simulink model "PitchHoldAndAirspeedHold"  (R2021b)
settings: Solver=VariableStepAuto  StartTime=0.0  StopTime=100  RelTol=1e-3
values from neighbouring files (symbols this model uses):
  alpha0 = 0.1824    [Glideslope.m]
  max_dev_elevator = 25 - trim_control_lo(1)    [Glideslope.m]
  max_dev_thrust = 19000 - trim_thrust_lo    [Glideslope.m]
  min_dev_elevator = -25 - trim_control_lo(1)    [Glideslope.m]
  min_dev_thrust = 1000 - trim_thrust_lo    [Glideslope.m]
  t0 = 10    [Glideslope.m]
  theta0 = 0.1824    [Glideslope.m]
  V_0 = 300    [Glideslope.m]
undefined symbols (not defined in the file or in its folder): coeff_x, coeff_y, magnitude, x0
libraries: slpidlib x3, cstblocks x1
settings Model: Creator=ddefu  LastModifiedBy=20181021

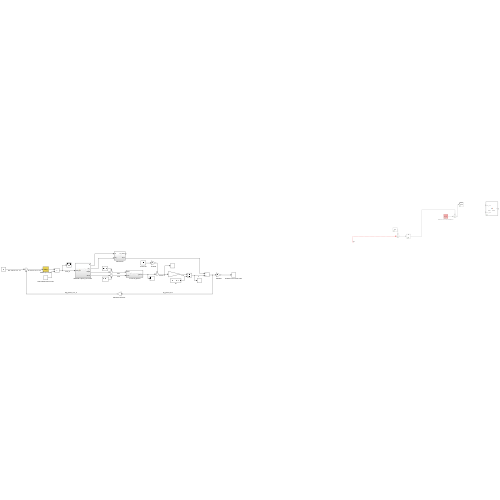
[thumbnail: Simulink's stored preview of the top-level diagram]
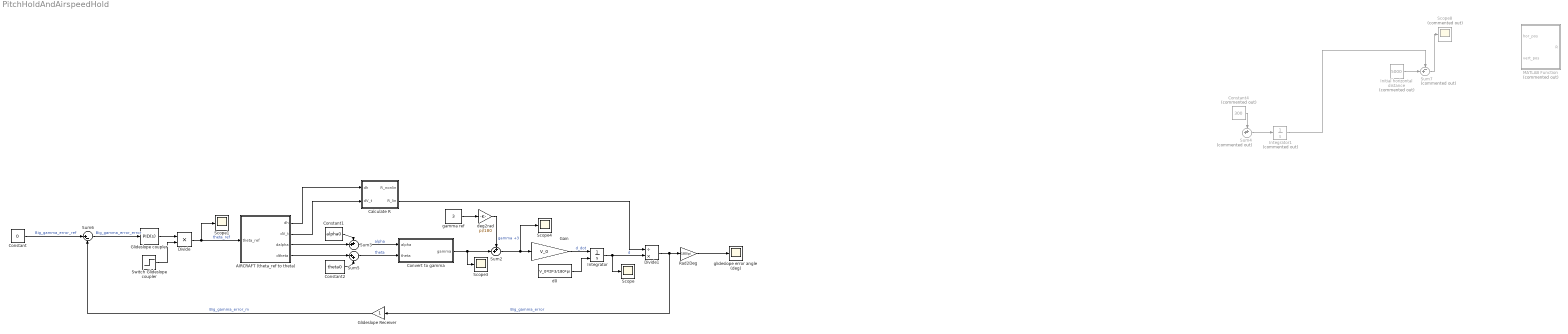
== system PitchHoldAndAirspeedHold ==
  AIRCRAFT (theta_ref to theta) : Subsystem
  Calculate R : Subsystem
  Constant : Constant  Value=0
  Constant1 : Constant  Value=alpha0
  Constant2 : Constant  Value=theta0
  Constant4 : Constant  Commented=on  Value=300
  Convert to gamma : Subsystem
  Divide : Product  Inputs=**
  Divide1 : Product  Inputs=/*
  Gain : Gain  Gain=V_0
  Glideslope Receiver : Gain
  Glideslope coupler : slpidlib/PID Controller  Controller=PID  Form=Parallel  TimeDomain=Continuous-time  UseExternalTs=off  SampleTime=-1  IntegratorMethod=Forward Euler  FilterMethod=Forward Euler  ControllerParametersSource=internal  P=100  I=10  D=0  UseFilter=on  N=100  TunerSelectOption=Transfer Function Based (PID Tuner App)  InitialConditionSource=internal  InitialConditionForIntegrator=0  InitialConditionForFilter=0  DifferentiatorICPrevScaledInput=0  ExternalReset=none  TrackingMode=off  Kt=1  LimitOutput=off  SatLimitsSource=internal  UpperSaturationLimit=inf  LowerSaturationLimit=-inf  LinearizeAsGain=on  AntiWindupMode=none  Kb=1  POutMin=[]  POutMax=[]  IOutMin=[]  IOutMax=[]  DOutMin=[]  DOutMax=[]  NOutMin=[]  NOutMax=[]  SumOutMin=[]  SumOutMax=[]  SaturationOutMin=[]  SaturationOutMax=[]  PParamMin=[]  PParamMax=[]  IParamMin=[]  IParamMax=[]  DParamMin=[]  DParamMax=[]  NParamMin=[]  NParamMax=[]  KbParamMin=[]  KbParamMax=[]  KtParamMin=[]  KtParamMax=[]  KbOutMin=[]  KbOutMax=[]  KtOutMin=[]  KtOutMax=[]  IntegratorOutMin=[]  IntegratorOutMax=[]  FilterOutMin=[]  FilterOutMax=[]  SumI1OutMin=[]  SumI1OutMax=[]  SumI2OutMin=[]  SumI2OutMax=[]  SumI3OutMin=[]  SumI3OutMax=[]  SumI4OutMin=[]  SumI4OutMax=[]  SumDOutMin=[]  SumDOutMax=[]  DifferentiatorOutMin=[]  DifferentiatorOutMax=[]  FilterDiffOutCoefMin=[]  FilterDiffOutCoefMax=[]  ReciprocalOutMin=[]  ReciprocalOutMax=[]  SumDenOutMin=[]  SumDenOutMax=[]  SumNumOutMin=[]  SumNumOutMax=[]  DivideOutMin=[]  DivideOutMax=[]  UdiffTsProdOutMin=[]  UdiffTsProdOutMax=[]  NTsProdOutMin=[]  NTsProdOutMax=[]  UintegralTsProdOutMin=[]  UintegralTsProdOutMax=[]  UngainTsProdOutMin=[]  UngainTsProdOutMax=[]  IntegratorContinuousStateAttributes=''  IntegratorStateMustResolveToSignalObject=off  IntegratorRTWStateStorageClass=Auto  FilterContinuousStateAttributes=''  FilterStateMustResolveToSignalObject=off  FilterRTWStateStorageClass=Auto  ParallelPVariant=InternalParameters  IdealPVariant=Disabled  IVariant=InternalParameters  DVariant=InternalParameters  IntegratorVariant=Continuous  SatVariant=Disabled  AWVariant=Passthrough  PCopyVariant=Disabled  TRVariant=Disabled  FdbkBlocksVariant=Forward  IdealPFdbkVariant=Disabled  SatFdbkVariant=Disabled  DerivativeFilterVariant=ContFilter  NVariant=InternalParameters  NCopyVariant=Disabled  FilterICVariant=InternalICsFilter  IntegratorICVariant=InternalICs  ExternalResetVariant=Disabled  TRSumVariant=Passthrough  SumFdbkVariant=Disabled  SumVariant=Sum_PID  TsampFilterVariant=InternalTs  TsampNgainVariant=Passthrough  TsampIntegralVariant=Passthrough  ExternalSaturationOutDataTypeStr=Inherit: Same as second input
  Initial horizontal distance : Constant  Commented=on  Value=5000
  Integrator : Integrator  InitialConditionSource=external
  Integrator1 : Integrator  Commented=on
  MATLAB Function : MATLAB Function  Commented=on  TreatAsAtomicUnit=on
  Rad2Deg : Gain  Gain=180/pi
  Scope{,1,3..4} (4 alike) : Scope
  Scope8 : Scope  Commented=on
  Sum2 : Sum  Inputs=++|
  Sum3 : Sum  Inputs=++|
  Sum4 : Sum  Commented=on  Inputs=++|
  Sum5 : Sum  Inputs=|++
  Sum6 : Sum  Inputs=|+-
  Sum7 : Sum  Commented=on  Inputs=-+|
  Switch Glideslope coupler : Step  Time=10  SampleTime=0
  d0 : Constant  Value=V_0*t0*3/180*pi
  deg2rad : Gain  Gain=pi/180
  gamma ref : Constant  Value=3
  glideslope error angle (deg) : Scope
  wires:
  Sum2/1 -> Scope4/1, Gain/1  "gamma +3"
  Gain/1 -> Integrator/1  "d_dot"
  Integrator/1 -> Divide1/2, Scope/1  "d"
  Convert to gamma/1(gamma) -> Sum2/2, Scope3/1
  Sum3/1 -> Convert to gamma/1(alpha)  "alpha"
  Constant1/1 -> Sum3/1
  Sum5/1 -> Convert to gamma/2(theta)  "theta"
  Divide1/1 -> Glideslope Receiver/1, Rad2Deg/1  "Big_gamma_error"
  Glideslope Receiver/1 -> Sum6/2  "Big_gamma_error_m"
  Constant/1 -> Sum6/1  "Big_gamma_error_ref"
  Sum6/1 -> Glideslope coupler/1  "Big_gamma_error_error"
  d0/1 -> Integrator/2
  Sum7/1 -> Scope8/1
  ? -> Sum4/2  "V_t"
  Integrator1/1 -> Sum7/1
  Constant4/1 -> Sum4/1
  Initial horizontal distance/1 -> Sum7/2
  Sum4/1 -> Integrator1/1
  Rad2Deg/1 -> glideslope error angle (deg)/1
  AIRCRAFT (theta_ref to theta)/1(dh) -> Calculate R/1(dh)
  AIRCRAFT (theta_ref to theta)/2(dV_t) -> Calculate R/2(dV_t)
  AIRCRAFT (theta_ref to theta)/3(dalpha) -> Sum3/2
  Switch Glideslope coupler/1 -> Divide/2
  Glideslope coupler/1 -> Divide/1
  Divide/1 -> Scope1/1, AIRCRAFT (theta_ref to theta)/1(theta_ref)  "theta_ref"
  Calculate R/2(R_lin) -> Divide1/1
  Constant2/1 -> Sum5/2
  AIRCRAFT (theta_ref to theta)/4(dtheta) -> Sum5/1
  gamma ref/1 -> deg2rad/1
  deg2rad/1 -> Sum2/1

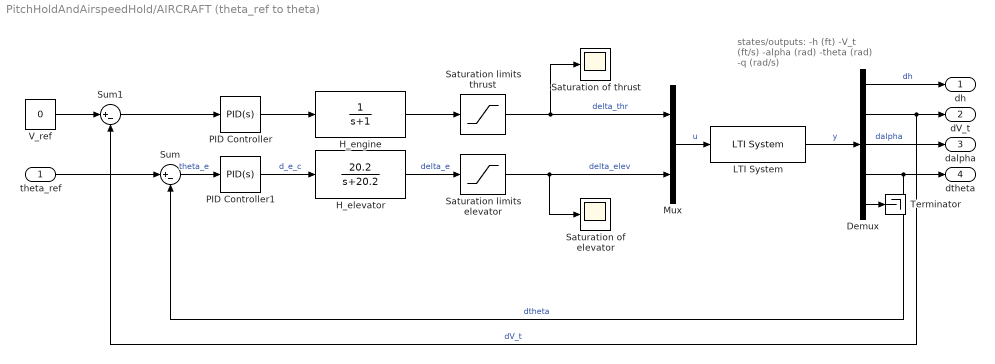
== system PitchHoldAndAirspeedHold/AIRCRAFT (theta_ref to theta) ==
  note: states/outputs:
      | -h (ft)
      | -V_t (ft/s)
      | -alpha (rad)
      | -theta (rad)
      | -q (rad/s)
  theta_ref : Inport
  Demux : Demux  Outputs=5
  H_elevator : TransferFcn  Numerator=[20.2]  Denominator=[1 20.2]
  H_engine : TransferFcn  Denominator=[1 1]
  LTI System : cstblocks/LTI System  sys=sys_reduced  IC=[0;0;0;0;0]
  Mux : Mux  Inputs=2
  PID Controller : slpidlib/PID Controller  Controller=PID  Form=Parallel  TimeDomain=Continuous-time  UseExternalTs=off  SampleTime=-1  IntegratorMethod=Forward Euler  FilterMethod=Forward Euler  ControllerParametersSource=internal  P=210  I=6  D=0  UseFilter=on  N=100  TunerSelectOption=Transfer Function Based (PID Tuner App)  InitialConditionSource=internal  InitialConditionForIntegrator=0  InitialConditionForFilter=0  DifferentiatorICPrevScaledInput=0  ExternalReset=none  TrackingMode=off  Kt=1  LimitOutput=off  SatLimitsSource=internal  UpperSaturationLimit=inf  LowerSaturationLimit=-inf  LinearizeAsGain=on  AntiWindupMode=none  Kb=1  POutMin=[]  POutMax=[]  IOutMin=[]  IOutMax=[]  DOutMin=[]  DOutMax=[]  NOutMin=[]  NOutMax=[]  SumOutMin=[]  SumOutMax=[]  SaturationOutMin=[]  SaturationOutMax=[]  PParamMin=[]  PParamMax=[]  IParamMin=[]  IParamMax=[]  DParamMin=[]  DParamMax=[]  NParamMin=[]  NParamMax=[]  KbParamMin=[]  KbParamMax=[]  KtParamMin=[]  KtParamMax=[]  KbOutMin=[]  KbOutMax=[]  KtOutMin=[]  KtOutMax=[]  IntegratorOutMin=[]  IntegratorOutMax=[]  FilterOutMin=[]  FilterOutMax=[]  SumI1OutMin=[]  SumI1OutMax=[]  SumI2OutMin=[]  SumI2OutMax=[]  SumI3OutMin=[]  SumI3OutMax=[]  SumI4OutMin=[]  SumI4OutMax=[]  SumDOutMin=[]  SumDOutMax=[]  DifferentiatorOutMin=[]  DifferentiatorOutMax=[]  FilterDiffOutCoefMin=[]  FilterDiffOutCoefMax=[]  ReciprocalOutMin=[]  ReciprocalOutMax=[]  SumDenOutMin=[]  SumDenOutMax=[]  SumNumOutMin=[]  SumNumOutMax=[]  DivideOutMin=[]  DivideOutMax=[]  UdiffTsProdOutMin=[]  UdiffTsProdOutMax=[]  NTsProdOutMin=[]  NTsProdOutMax=[]  UintegralTsProdOutMin=[]  UintegralTsProdOutMax=[]  UngainTsProdOutMin=[]  UngainTsProdOutMax=[]  IntegratorContinuousStateAttributes=''  IntegratorStateMustResolveToSignalObject=off  IntegratorRTWStateStorageClass=Auto  FilterContinuousStateAttributes=''  FilterStateMustResolveToSignalObject=off  FilterRTWStateStorageClass=Auto  ParallelPVariant=InternalParameters  IdealPVariant=Disabled  IVariant=InternalParameters  DVariant=InternalParameters  IntegratorVariant=Continuous  SatVariant=Disabled  AWVariant=Passthrough  PCopyVariant=Disabled  TRVariant=Disabled  FdbkBlocksVariant=Forward  IdealPFdbkVariant=Disabled  SatFdbkVariant=Disabled  DerivativeFilterVariant=ContFilter  NVariant=InternalParameters  NCopyVariant=Disabled  FilterICVariant=InternalICsFilter  IntegratorICVariant=InternalICs  ExternalResetVariant=Disabled  TRSumVariant=Passthrough  SumFdbkVariant=Disabled  SumVariant=Sum_PID  TsampFilterVariant=InternalTs  TsampNgainVariant=Passthrough  TsampIntegralVariant=Passthrough  ExternalSaturationOutDataTypeStr=Inherit: Same as second input
  PID Controller1 : slpidlib/PID Controller  Controller=PID  Form=Parallel  TimeDomain=Continuous-time  UseExternalTs=off  SampleTime=-1  IntegratorMethod=Forward Euler  FilterMethod=Forward Euler  ControllerParametersSource=internal  P=-100  I=-10  D=-70  UseFilter=on  N=100  TunerSelectOption=Transfer Function Based (PID Tuner App)  InitialConditionSource=internal  InitialConditionForIntegrator=0  InitialConditionForFilter=0  DifferentiatorICPrevScaledInput=0  ExternalReset=none  TrackingMode=off  Kt=1  LimitOutput=off  SatLimitsSource=internal  UpperSaturationLimit=inf  LowerSaturationLimit=-inf  LinearizeAsGain=on  AntiWindupMode=none  Kb=1  POutMin=[]  POutMax=[]  IOutMin=[]  IOutMax=[]  DOutMin=[]  DOutMax=[]  NOutMin=[]  NOutMax=[]  SumOutMin=[]  SumOutMax=[]  SaturationOutMin=[]  SaturationOutMax=[]  PParamMin=[]  PParamMax=[]  IParamMin=[]  IParamMax=[]  DParamMin=[]  DParamMax=[]  NParamMin=[]  NParamMax=[]  KbParamMin=[]  KbParamMax=[]  KtParamMin=[]  KtParamMax=[]  KbOutMin=[]  KbOutMax=[]  KtOutMin=[]  KtOutMax=[]  IntegratorOutMin=[]  IntegratorOutMax=[]  FilterOutMin=[]  FilterOutMax=[]  SumI1OutMin=[]  SumI1OutMax=[]  SumI2OutMin=[]  SumI2OutMax=[]  SumI3OutMin=[]  SumI3OutMax=[]  SumI4OutMin=[]  SumI4OutMax=[]  SumDOutMin=[]  SumDOutMax=[]  DifferentiatorOutMin=[]  DifferentiatorOutMax=[]  FilterDiffOutCoefMin=[]  FilterDiffOutCoefMax=[]  ReciprocalOutMin=[]  ReciprocalOutMax=[]  SumDenOutMin=[]  SumDenOutMax=[]  SumNumOutMin=[]  SumNumOutMax=[]  DivideOutMin=[]  DivideOutMax=[]  UdiffTsProdOutMin=[]  UdiffTsProdOutMax=[]  NTsProdOutMin=[]  NTsProdOutMax=[]  UintegralTsProdOutMin=[]  UintegralTsProdOutMax=[]  UngainTsProdOutMin=[]  UngainTsProdOutMax=[]  IntegratorContinuousStateAttributes=''  IntegratorStateMustResolveToSignalObject=off  IntegratorRTWStateStorageClass=Auto  FilterContinuousStateAttributes=''  FilterStateMustResolveToSignalObject=off  FilterRTWStateStorageClass=Auto  ParallelPVariant=InternalParameters  IdealPVariant=Disabled  IVariant=InternalParameters  DVariant=InternalParameters  IntegratorVariant=Continuous  SatVariant=Disabled  AWVariant=Passthrough  PCopyVariant=Disabled  TRVariant=Disabled  FdbkBlocksVariant=Forward  IdealPFdbkVariant=Disabled  SatFdbkVariant=Disabled  DerivativeFilterVariant=ContFilter  NVariant=InternalParameters  NCopyVariant=Disabled  FilterICVariant=InternalICsFilter  IntegratorICVariant=InternalICs  ExternalResetVariant=Disabled  TRSumVariant=Passthrough  SumFdbkVariant=Disabled  SumVariant=Sum_PID  TsampFilterVariant=InternalTs  TsampNgainVariant=Passthrough  TsampIntegralVariant=Passthrough  ExternalSaturationOutDataTypeStr=Inherit: Same as second input
  Saturation limits elevator : Saturate  UpperLimit=max_dev_elevator  LowerLimit=min_dev_elevator
  Saturation limits thrust : Saturate  UpperLimit=max_dev_thrust  LowerLimit=min_dev_thrust
  Saturation of elevator : Scope
  Saturation of thrust : Scope
  Sum : Sum  Inputs=|+-
  Sum1 : Sum  Inputs=|+-
  Terminator : Terminator
  V_ref : Constant  Value=0
  dh : Outport
  dV_t : Outport  Port=2
  dalpha : Outport  Port=3
  dtheta : Outport  Port=4
  wires:
  Saturation limits thrust/1 -> Saturation of thrust/1, Mux/1  "delta_thr"
  Demux/2 -> Sum1/2, dV_t/1  "dV_t"
  Demux/4 -> Sum/2, dtheta/1  "dtheta"
  Demux/1 -> dh/1  "dh"
  Demux/3 -> dalpha/1  "dalpha"
  Saturation limits elevator/1 -> Saturation of elevator/1, Mux/2  "delta_elev"
  V_ref/1 -> Sum1/1
  H_elevator/1 -> Saturation limits elevator/1  "delta_e"
  PID Controller/1 -> H_engine/1
  H_engine/1 -> Saturation limits thrust/1
  PID Controller1/1 -> H_elevator/1  "d_e_c"
  LTI System/1 -> Demux/1  "y"
  Mux/1 -> LTI System/1  "u"
  theta_ref/1 -> Sum/1
  Sum1/1 -> PID Controller/1
  Sum/1 -> PID Controller1/1  "theta_e"
  Demux/5 -> Terminator/1

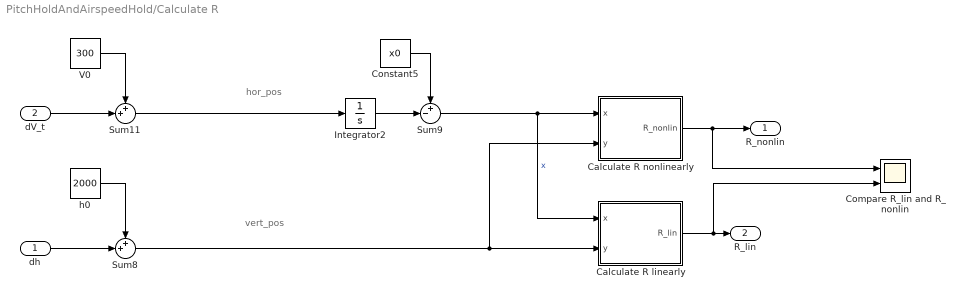
== system PitchHoldAndAirspeedHold/Calculate R ==
  note: vert_pos
  note: hor_pos
  dh : Inport
  dV_t : Inport  Port=2
  Calculate R linearly : Subsystem
  Calculate R nonlinearly : Subsystem
  Compare R_lin and R_nonlin : Scope  NumInputPorts=2
  Constant5 : Constant  Value=x0
  Integrator2 : Integrator
  Sum11 : Sum  Inputs=++|
  Sum8 : Sum  Inputs=++|
  Sum9 : Sum  Inputs=+-|
  V0 : Constant  Value=300
  h0 : Constant  Value=2000
  R_nonlin : Outport
  R_lin : Outport  Port=2
  wires:
  Sum8/1 -> Calculate R linearly/2(y), Calculate R nonlinearly/2(y)
  Sum9/1 -> Calculate R linearly/1(x), Calculate R nonlinearly/1(x)  "x"
  dh/1 -> Sum8/2
  dV_t/1 -> Sum11/2
  h0/1 -> Sum8/1
  Integrator2/1 -> Sum9/2
  Sum11/1 -> Integrator2/1
  Constant5/1 -> Sum9/1
  V0/1 -> Sum11/1
  Calculate R linearly/1(R_lin) -> Compare R_lin and R_nonlin/2, R_lin/1
  Calculate R nonlinearly/1(R_nonlin) -> Compare R_lin and R_nonlin/1, R_nonlin/1

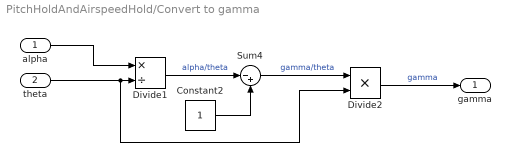
== system PitchHoldAndAirspeedHold/Convert to gamma ==
  alpha : Inport
  theta : Inport  Port=2
  Constant2 : Constant
  Divide1 : Product  Inputs=*/
  Divide2 : Product  Inputs=**
  Sum4 : Sum  Inputs=|-+
  gamma : Outport
  wires:
  Divide1/1 -> Sum4/1  "alpha/theta"
  Sum4/1 -> Divide2/1  "gamma/theta"
  Constant2/1 -> Sum4/2
  Divide2/1 -> gamma/1  "gamma"
  alpha/1 -> Divide1/1
  theta/1 -> Divide2/2, Divide1/2

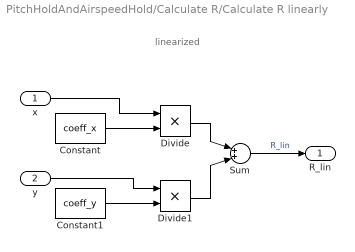
== system PitchHoldAndAirspeedHold/Calculate R/Calculate R linearly ==
  note: linearized
  x : Inport
  y : Inport  Port=2
  Constant : Constant  Value=coeff_x
  Constant1 : Constant  Value=coeff_y
  Divide : Product  Inputs=**
  Divide1 : Product  Inputs=**
  Sum : Sum  Inputs=|++|
  R_lin : Outport
  wires:
  y/1 -> Divide1/1
  Constant1/1 -> Divide1/2
  Divide/1 -> Sum/1
  Divide1/1 -> Sum/2
  Constant/1 -> Divide/2
  Sum/1 -> R_lin/1  "R_lin"
  x/1 -> Divide/1

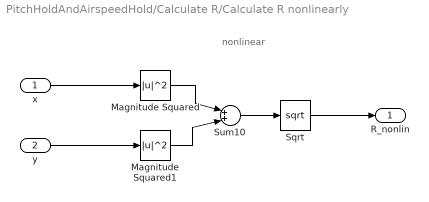
== system PitchHoldAndAirspeedHold/Calculate R/Calculate R nonlinearly ==
  note: nonlinear
  x : Inport
  y : Inport  Port=2
  Magnitude Squared : Math  Operator=magnitude^2  SaturateOnIntegerOverflow=on
  Magnitude Squared1 : Math  Operator=magnitude^2  SaturateOnIntegerOverflow=on
  Sqrt : Sqrt  SaturateOnIntegerOverflow=on
  Sum10 : Sum  Inputs=|++|
  R_nonlin : Outport
  wires:
  Magnitude Squared/1 -> Sum10/1
  Magnitude Squared1/1 -> Sum10/2
  Sum10/1 -> Sqrt/1
  Sqrt/1 -> R_nonlin/1
  x/1 -> Magnitude Squared/1
  y/1 -> Magnitude Squared1/1

== matlab function PitchHoldAndAirspeedHold/MATLAB Function ==
  data: hor_pos input; R output; vert_pos input
function R = slant_range(hor_pos, vert_pos)

R = sqrt(hor_pos^2+vert_pos^2);
